simulink model "controller_v10"  (R2020b)
settings: Solver=FixedStepDiscrete  StartTime=0.0  StopTime=inf  RelTol=1e-3
undefined symbols (not defined in the file): ctr, DiscIntNeverNeededParam, flt, IO397, mdl, rbt, rsim, som
libraries: simulink x30, slrealtimeloglib x12, slrealtimeseriallib x5, slrealtimetgmanagement x4, speedgoatlib_fpga_analog_io x4, speedgoatlib_fpga x2, dspfdesign x1, speedgoatlib_fpga_dio x1, slrealtimeutilitieslib x1
(part 2 of 2)

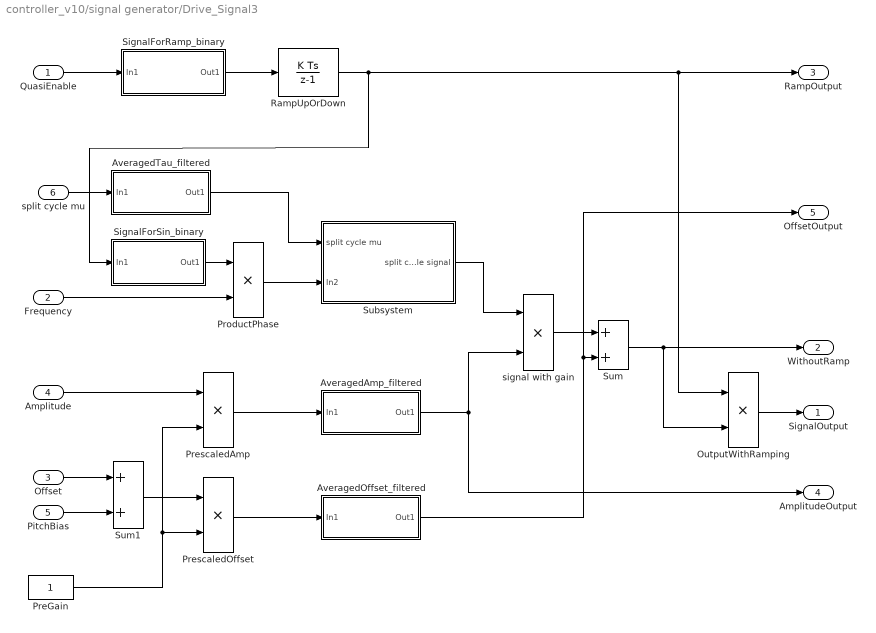
== system controller_v10/signal generator/Drive_Signal3 ==
  QuasiEnable : Inport
  Frequency : Inport  Port=2
  Offset : Inport  Port=3
  Amplitude : Inport  Port=4
  PitchBias : Inport  Port=5
  split cycle mu : Inport  Port=6
  AveragedAmp_filtered : Subsystem
  AveragedOffset_filtered : Subsystem
  AveragedTau_filtered : Subsystem
  OutputWithRamping : Product  RndMeth=Zero
  PreGain : Constant
  PrescaledAmp : Product  RndMeth=Zero
  PrescaledOffset : Product  RndMeth=Zero
  ProductPhase : Product  RndMeth=Zero
  RampUpOrDown : DiscreteIntegrator  gainval=10  SampleTime=-1  LimitOutput=on  UpperSaturationLimit=1  LowerSaturationLimit=0  ICPrevOutput=DiscIntNeverNeededParam  ICPrevScaledInput=DiscIntNeverNeededParam
  SignalForRamp_binary : Subsystem
  SignalForSin_binary : Subsystem
  Subsystem : Subsystem
  Sum : Sum
  Sum1 : Sum
  signal with gain : Product  RndMeth=Zero
  SignalOutput : Outport
  WithoutRamp : Outport  Port=2
  RampOutput : Outport  Port=3
  AmplitudeOutput : Outport  Port=4
  OffsetOutput : Outport  Port=5
  wires:
  PrescaledAmp/1 -> AveragedAmp_filtered/1(In1)
  Sum/1 -> OutputWithRamping/2, WithoutRamp/1
  RampUpOrDown/1 -> RampOutput/1, OutputWithRamping/1, SignalForSin_binary/1(In1)
  QuasiEnable/1 -> SignalForRamp_binary/1(In1)
  SignalForRamp_binary/1(Out1) -> RampUpOrDown/1
  Amplitude/1 -> PrescaledAmp/1
  signal with gain/1 -> Sum/1
  Frequency/1 -> ProductPhase/2
  SignalForSin_binary/1(Out1) -> ProductPhase/1
  ProductPhase/1 -> Subsystem/2(In2)
  AveragedOffset_filtered/1(Out1) -> Sum/2, OffsetOutput/1
  PrescaledOffset/1 -> AveragedOffset_filtered/1(In1)
  PreGain/1 -> PrescaledAmp/2, PrescaledOffset/2
  OutputWithRamping/1 -> SignalOutput/1
  AveragedAmp_filtered/1(Out1) -> signal with gain/2, AmplitudeOutput/1
  Sum1/1 -> PrescaledOffset/1
  Offset/1 -> Sum1/1
  PitchBias/1 -> Sum1/2
  AveragedTau_filtered/1(Out1) -> Subsystem/1(split cycle mu)
  split cycle mu/1 -> AveragedTau_filtered/1(In1)
  Subsystem/1(split cycle signal) -> signal with gain/1

== system controller_v10/signal generator/SignalSaturationLimit ==
  BiasMax : Inport
  SignalRaw : Inport  Port=2
  GainBias : Gain
  MaxOf : MinMax  Function=max  Inputs=2
  MinOf : MinMax  Inputs=2
  ground : Constant
  SignalSatd : Outport
  wires:
  BiasMax/1 -> GainBias/1
  SignalRaw/1 -> MinOf/2
  MinOf/1 -> MaxOf/1
  MaxOf/1 -> SignalSatd/1
  GainBias/1 -> MinOf/1
  ground/1 -> MaxOf/2

== system controller_v10/signal generator/SignalSaturationLimit1 ==
  BiasMax : Inport
  SignalRaw : Inport  Port=2
  GainBias : Gain
  MaxOf : MinMax  Function=max  Inputs=2
  MinOf : MinMax  Inputs=2
  ground : Constant
  SignalSatd : Outport
  wires:
  BiasMax/1 -> GainBias/1
  SignalRaw/1 -> MinOf/2
  MinOf/1 -> MaxOf/1
  MaxOf/1 -> SignalSatd/1
  GainBias/1 -> MinOf/1
  ground/1 -> MaxOf/2

== system controller_v10/signal generator/SignalSaturationLimit2 ==
  BiasMax : Inport
  SignalRaw : Inport  Port=2
  GainBias : Gain
  MaxOf : MinMax  Function=max  Inputs=2
  MinOf : MinMax  Inputs=2
  ground : Constant
  SignalSatd : Outport
  wires:
  BiasMax/1 -> GainBias/1
  SignalRaw/1 -> MinOf/2
  MinOf/1 -> MaxOf/1
  MaxOf/1 -> SignalSatd/1
  GainBias/1 -> MinOf/1
  ground/1 -> MaxOf/2

== system controller_v10/signal generator/SignalSaturationLimit3 ==
  BiasMax : Inport
  SignalRaw : Inport  Port=2
  GainBias : Gain
  MaxOf : MinMax  Function=max  Inputs=2
  MinOf : MinMax  Inputs=2
  ground : Constant
  SignalSatd : Outport
  wires:
  BiasMax/1 -> GainBias/1
  SignalRaw/1 -> MinOf/2
  MinOf/1 -> MaxOf/1
  MaxOf/1 -> SignalSatd/1
  GainBias/1 -> MinOf/1
  ground/1 -> MaxOf/2

== system controller_v10/Adaptive Controller/adaptive system/integrator ==
  note: integrator limit (saturation) needs to be set.
  e : Inport
  torque offset : Inport  Port=2
  thrust_offset : Inport  Port=3
  enable1 : Product  Inputs=**
  initial guess : MATLAB Function  TreatAsAtomicUnit=on
  integrator with sat : DiscreteIntegrator  IntegratorMethod=Integration: Backward Euler  gainval=1  SampleTime=-1  LimitOutput=on  UpperSaturationLimit=ctr.integral.lim.upper  LowerSaturationLimit=ctr.integral.lim.lower  ICPrevOutput=DiscIntNeverNeededParam  ICPrevScaledInput=DiscIntNeverNeededParam
  safety2 : Subsystem
  start ramp : Subsystem
  int_e : Outport
  " torq_off" : Outport  Port=2
  th_off : Outport  Port=3
  wires:
  safety2/1(Out1) -> enable1/2
  enable1/1 -> integrator with sat/1
  start ramp/1(Out1) -> enable1/1
  e/1 -> safety2/1(In1)
  integrator with sat/1 -> initial guess/1(i_e)
  initial guess/1(int_e) -> int_e/1
  initial guess/2(tor_inte) -> " torq_off"/1
  initial guess/3(th_inte) -> th_off/1
  torque offset/1 -> initial guess/2(tor_off)
  thrust_offset/1 -> initial guess/3(th_off)

== system controller_v10/Adaptive Controller/adaptive system/safety1 ==
  In1 : Inport
  Compare To Constant1 : simulink/Logic and Bit Operations/Compare To Constant  relop=<=  const=inf  OutDataTypeStr=uint8
  Switch1 : Switch  Threshold=0.5
  zero1 : Constant  Value=0
  Out1 : Outport
  wires:
  In1/1 -> Switch1/1, Compare To Constant1/1
  Compare To Constant1/1 -> Switch1/2
  zero1/1 -> Switch1/3
  Switch1/1 -> Out1/1

== system controller_v10/Adaptive Controller/adaptive system/safety2 ==
  In1 : Inport
  Compare To Constant1 : simulink/Logic and Bit Operations/Compare To Constant  relop=<=  const=inf  OutDataTypeStr=uint8
  Switch1 : Switch  Threshold=0.5
  zero1 : Constant  Value=0
  Out1 : Outport
  wires:
  In1/1 -> Switch1/1, Compare To Constant1/1
  Compare To Constant1/1 -> Switch1/2
  zero1/1 -> Switch1/3
  Switch1/1 -> Out1/1

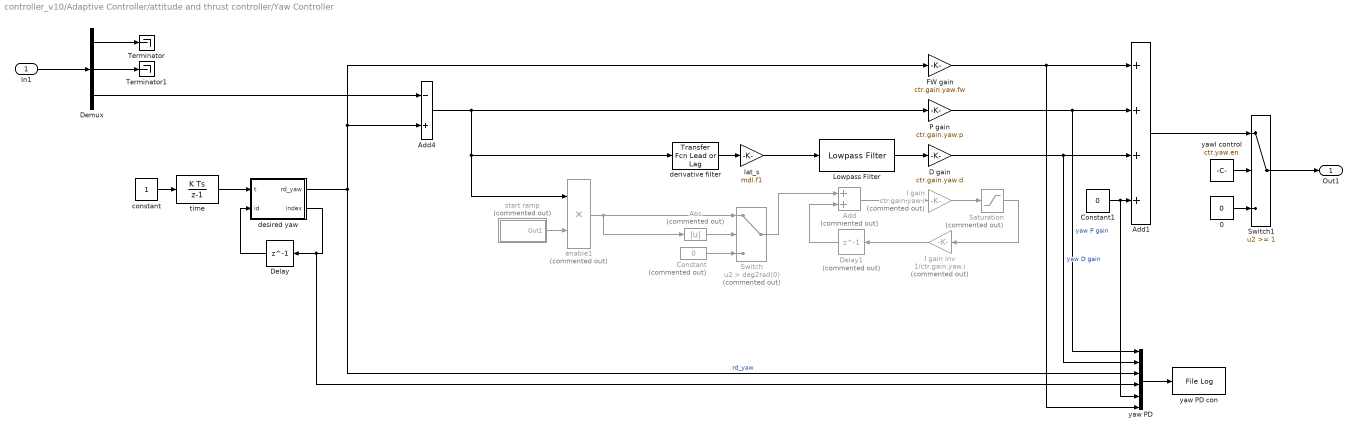
== system controller_v10/Adaptive Controller/attitude and thrust controller/Yaw Controller ==
  In1 : Inport
  0 : Constant  Value=0  SampleTime=-1
  Abs : Abs  Commented=on
  Add : Sum  Commented=on
  Add1 : Sum  Inputs=++++
  Add4 : Sum  Inputs=-+
  Constant : Constant  Commented=on  Value=0
  Constant1 : Constant  Value=0  SampleTime=-1
  D gain : Gain  Gain=ctr.gain.yaw.d
  Delay : Delay  DelayLength=1  InitialCondition=1
  Delay1 : Delay  Commented=on  DelayLength=1
  Demux : Demux  Outputs=3
  FW gain : Gain  Gain=ctr.gain.yaw.fw
  I gain : Gain  Commented=on  Gain=ctr.gain.yaw.i
  I gain inv : Gain  Commented=on  Gain=1/ctr.gain.yaw.i
  Lowpass Filter : dspfdesign/Lowpass Filter  FilterType=FIR  DesignForMinimumOrder=on  FilterOrder=2000  PassbandFrequency=7  StopbandFrequency=90  PassbandRipple=0.5  StopbandAttenuation=75  InheritSampleRate=off  SampleRate=10000  SimulateUsing=Interpreted execution  roundingMode=Floor  coeffsDataTypeStr=fixdt(1,16)
  P gain : Gain  Gain=ctr.gain.yaw.p
  Saturation : Saturate  Commented=on  UpperLimit=ctr.integral.yaw.upper  LowerLimit=ctr.integral.yaw.lower
  Switch : Switch  Commented=on  Criteria=u2 > Threshold  Threshold=deg2rad(0)
  Switch1 : Switch  Threshold=1
  Terminator : Terminator
  Terminator1 : Terminator
  constant : Constant
  derivative filter : simulink/Discrete/Transfer Fcn Lead or Lag  PoleZ=mdl.zf1  ZeroZ=1  ICPrevOutput=0.0  ICPrevInput=0.0  DoSatur=off
      settings: SourceProductBaseCode=SL
  desired yaw : MATLAB Function  TreatAsAtomicUnit=on
  enable1 : Product  Commented=on  Inputs=**
  lat_s : Gain  Gain=mdl.f1
  start ramp : Subsystem  Commented=on
  time : DiscreteIntegrator  gainval=1  SampleTime=-1  UpperSaturationLimit=1  LowerSaturationLimit=0  ICPrevOutput=DiscIntNeverNeededParam  ICPrevScaledInput=DiscIntNeverNeededParam
  yaw PD : Mux  Inputs=6
  yaw PD con : slrealtimeloglib/File Log  decimation=1
      settings: SourceProductBaseCode=XP
  yawl control : Constant  Value=ctr.yaw.en
  Out1 : Outport
  wires:
  Demux/1 -> Terminator/1
  Demux/2 -> Terminator1/1
  Demux/3 -> Add4/1
  0/1 -> Switch1/3
  yawl control/1 -> Switch1/2
  In1/1 -> Demux/1
  Add4/1 -> P gain/1, enable1/1, derivative filter/1
  Switch1/1 -> Out1/1
  derivative filter/1 -> lat_s/1
  Add1/1 -> Switch1/1
  P gain/1 -> yaw PD/1, Add1/2  "yaw P gain"
  D gain/1 -> yaw PD/2, Add1/3  "yaw D gain"
  yaw PD/1 -> yaw PD con/1
  Lowpass Filter/1 -> D gain/1
  lat_s/1 -> Lowpass Filter/1
  constant/1 -> time/1
  time/1 -> desired yaw/1(t)
  desired yaw/1(rd_yaw) -> FW gain/1, Add4/2, yaw PD/3  "rd_yaw"
  desired yaw/2(index) -> yaw PD/4, Delay/1
  Delay/1 -> desired yaw/2(id)
  Saturation/1 -> I gain inv/1
  I gain/1 -> Saturation/1
  enable1/1 -> Switch/1, Abs/1
  Delay1/1 -> Add/2
  Add/1 -> I gain/1
  I gain inv/1 -> Delay1/1
  start ramp/1(Out1) -> enable1/2
  Constant/1 -> Switch/3
  Switch/1 -> Add/1
  Abs/1 -> Switch/2
  FW gain/1 -> yaw PD/6, Add1/1
  Constant1/1 -> yaw PD/5, Add1/4

== system controller_v10/Adaptive Controller/observer/Rotaion ==
  Euler : Inport
  Rotation Matrix : MATLAB Function  TreatAsAtomicUnit=on
  Rotation Matrix1 : MATLAB Function  TreatAsAtomicUnit=on
  filtered derivative : Subsystem
  R : Outport
  Rdot : Outport  Port=2
  Omega : Outport  Port=3
  wires:
  Rotation Matrix/1(R) -> filtered derivative/1(In1), Rotation Matrix1/1(R), R/1
  Euler/1 -> Rotation Matrix/1(euler_angles)
  filtered derivative/1(Out1) -> Rotation Matrix1/2(Rdot), Rdot/1
  Rotation Matrix1/1(w) -> Omega/1

== system controller_v10/Adaptive Controller/observer/lateral observer ==
  XYZ : Inport
  derivative filter : simulink/Discrete/Transfer Fcn Lead or Lag  PoleZ=mdl.zf1  ZeroZ=1  ICPrevOutput=0.0  ICPrevInput=0.0  DoSatur=off
      settings: SourceProductBaseCode=SL
  derivative filter1 : simulink/Discrete/Transfer Fcn Lead or Lag  PoleZ=mdl.zf2  ZeroZ=1  ICPrevOutput=0.0  ICPrevInput=0.0  DoSatur=off
      settings: SourceProductBaseCode=SL
  derivative filter2 : simulink/Discrete/Transfer Fcn Lead or Lag  PoleZ=mdl.zf2  ZeroZ=1  ICPrevOutput=0.0  ICPrevInput=0.0  DoSatur=off
      settings: SourceProductBaseCode=SL
  lat_s : Gain  Gain=mdl.f1
  lat_s2 : Gain  Gain=mdl.f2
  lat_s2_ : Gain  Gain=mdl.f2
  saturation : Subsystem
  r : Outport
  r_dot : Outport  Port=2
  r_dotdot : Outport  Port=3
  wires:
  derivative filter1/1 -> derivative filter2/1
  derivative filter/1 -> lat_s/1
  XYZ/1 -> derivative filter/1, derivative filter1/1, r/1
  derivative filter2/1 -> lat_s2/1
  lat_s/1 -> r_dot/1
  lat_s2/1 -> lat_s2_/1
  lat_s2_/1 -> saturation/1(In1)
  saturation/1(Out1) -> r_dotdot/1

== system controller_v10/Force//Torque to Trajectory Specs/nominal desired voltage/force to voltage (hovering)  ==
  note: apply max voltage limit
  note: known correction from open-loop tests
  force : Inport
  Add : Sum  Inputs=+++
  Constant : Constant  Value=rbt.VM_input1
  Constant1 : Constant  Value=rbt.DV
  Constant2 : Constant  Value=rbt.VM_input2
  MATLAB Function : MATLAB Function  TreatAsAtomicUnit=on
  Product : Product
  Vout : Outport
  wires:
  MATLAB Function/1(Vo) -> Vout/1
  force/1 -> Product/2
  Constant2/1 -> Add/2
  Product/1 -> Add/3
  Add/1 -> MATLAB Function/1(Vi)
  Constant1/1 -> Add/1
  Constant/1 -> Product/1

== system controller_v10/Force//Torque to Trajectory Specs/nominal desired voltage/force to voltage flipping ==
  note: apply max voltage limit
  note: known correction from open-loop tests
  force : Inport
  Add : Sum
  Constant : Constant  Value=rbt.VM2
  Constant1 : Constant  Value=rbt.DV_flip
  MATLAB Function : MATLAB Function  TreatAsAtomicUnit=on
  Product : Product
  Sqrt : Sqrt  SaturateOnIntegerOverflow=on
  Vout : Outport
  wires:
  MATLAB Function/1(Vo) -> Vout/1
  force/1 -> Sqrt/1
  Add/1 -> MATLAB Function/1(Vi)
  Constant1/1 -> Add/1
  Constant/1 -> Product/1
  Product/1 -> Add/2
  Sqrt/1 -> Product/2

== system controller_v10/Measurement manager/safety check system/landing condition ==
  z : Inport
  Add : Sum  Inputs=+--
  SaturatingRamp1 : DiscreteIntegrator  gainval=1  SampleTime=-1  UpperSaturationLimit=1  LowerSaturationLimit=0  ICPrevOutput=DiscIntNeverNeededParam  ICPrevScaledInput=DiscIntNeverNeededParam
  constant : Constant
  constant1 : Constant  Value=2
  constant2 : Constant  Value=mdl.i_delay
  landing_cond : MATLAB Function  TreatAsAtomicUnit=on  SystemSampleTime=mdl.T
  en : Outport
  wires:
  SaturatingRamp1/1 -> Add/1
  constant/1 -> SaturatingRamp1/1
  constant1/1 -> Add/2
  constant2/1 -> Add/3
  Add/1 -> landing_cond/2(time_cond)
  z/1 -> landing_cond/1(alt)
  landing_cond/1(en) -> en/1

== system controller_v10/signal generator/Bias_Signal/AveragedBias ==
  note: To avoid having signal "jump",
      | we want SMOOTH transitions
      | in frequency (i.e., a weighted sum
      | of current freq and freq some delta t ago)
  note: time constant = 0.002sec
  In1 : Inport
  Discrete Transfer Fcn : DiscreteTransferFcn  Numerator=[0.05]  Denominator=[1 -.95]
  Out1 : Outport
  wires:
  In1/1 -> Discrete Transfer Fcn/1
  Discrete Transfer Fcn/1 -> Out1/1

== system controller_v10/signal generator/Bias_Signal/SIgnalForRamp_binary ==
  note: Should output 1 or -1,
      | so signal ramps UP to 1
      | or DOWN to 0.
  In1 : Inport
  Add : Sum  Inputs=+-
  Compare To Zero : simulink/Logic and Bit Operations/Compare To Zero  relop=>  OutDataTypeStr=uint8  ZeroCross=off
  Constant : Constant
  Data Type Conversion : DataTypeConversion  OutDataTypeStr=double
  Gain : Gain  Gain=2
  Out1 : Outport
  wires:
  In1/1 -> Compare To Zero/1
  Compare To Zero/1 -> Data Type Conversion/1
  Gain/1 -> Add/1
  Constant/1 -> Add/2
  Add/1 -> Out1/1
  Data Type Conversion/1 -> Gain/1

== system controller_v10/signal generator/Drive_Signal/AveragedAmp_filtered ==
  note: To avoid having signal "jump",
      | we want SMOOTH transitions
      | in frequency (i.e., a weighted sum
      | of current freq and freq some delta t ago)
  note: time constant 0.002sec
      | for 10kHz samping
  Amplitude : Inport
  Discrete Transfer Fcn : DiscreteTransferFcn  Numerator=[0.05]  Denominator=[1 -.95]
  Out1 : Outport
  wires:
  Amplitude/1 -> Discrete Transfer Fcn/1
  Discrete Transfer Fcn/1 -> Out1/1

== system controller_v10/signal generator/Drive_Signal/SignalForRamp_binary ==
  note: Should output 1 or -1,
      | so signal ramps UP to 1
      | or DOWN to 0.
  In1 : Inport
  Add : Sum  Inputs=+-
  Compare To Zero : simulink/Logic and Bit Operations/Compare To Zero  relop=>  OutDataTypeStr=uint8  ZeroCross=off
  Constant : Constant
  Data Type Conversion : DataTypeConversion  OutDataTypeStr=double
  Gain : Gain  Gain=2
  Out1 : Outport
  wires:
  In1/1 -> Compare To Zero/1
  Compare To Zero/1 -> Data Type Conversion/1
  Gain/1 -> Add/1
  Constant/1 -> Add/2
  Add/1 -> Out1/1
  Data Type Conversion/1 -> Gain/1

== system controller_v10/signal generator/Drive_Signal/SignalForSin_binary ==
  note: We want this to stay "high" for 1
      | second after the actual "enable"
      | is turned off...
  In1 : Inport
  Compare To Zero : simulink/Logic and Bit Operations/Compare To Zero  relop=>  OutDataTypeStr=uint8  ZeroCross=off
  Data Type Conversion : DataTypeConversion  OutDataTypeStr=double
  Out1 : Outport
  wires:
  In1/1 -> Compare To Zero/1
  Compare To Zero/1 -> Data Type Conversion/1
  Data Type Conversion/1 -> Out1/1

== system controller_v10/signal generator/Drive_Signal/Subsystem ==
  note: Amplitude compensation
      | keep the amplitude to be unity
  In2 : Inport
  2pi : Gain  Gain=2*pi
  Add : Sum
  deg to rad : Gain  Gain=pi/180
  first harmonic : Trigonometry  OutputSignalType=real
  omega*t : DiscreteIntegrator  SampleTime=-1  ICPrevOutput=DiscIntNeverNeededParam  ICPrevScaledInput=DiscIntNeverNeededParam
  phase offset : Constant  Value=0
  split cycle signal : Outport
  wires:
  first harmonic/1 -> split cycle signal/1
  In2/1 -> 2pi/1
  2pi/1 -> omega*t/1
  omega*t/1 -> Add/2
  Add/1 -> first harmonic/1
  phase offset/1 -> deg to rad/1
  deg to rad/1 -> Add/1

== system controller_v10/signal generator/Drive_Signal1/AveragedAmp_filtered ==
  note: To avoid having signal "jump",
      | we want SMOOTH transitions
      | in frequency (i.e., a weighted sum
      | of current freq and freq some delta t ago)
  note: time constant 0.002sec
      | for 10kHz samping
  Amplitude : Inport
  Discrete Transfer Fcn : DiscreteTransferFcn  Numerator=[0.05]  Denominator=[1 -.95]
  Out1 : Outport
  wires:
  Amplitude/1 -> Discrete Transfer Fcn/1
  Discrete Transfer Fcn/1 -> Out1/1

== system controller_v10/signal generator/Drive_Signal1/SignalForRamp_binary ==
  note: Should output 1 or -1,
      | so signal ramps UP to 1
      | or DOWN to 0.
  In1 : Inport
  Add : Sum  Inputs=+-
  Compare To Zero : simulink/Logic and Bit Operations/Compare To Zero  relop=>  OutDataTypeStr=uint8  ZeroCross=off
  Constant : Constant
  Data Type Conversion : DataTypeConversion  OutDataTypeStr=double
  Gain : Gain  Gain=2
  Out1 : Outport
  wires:
  In1/1 -> Compare To Zero/1
  Compare To Zero/1 -> Data Type Conversion/1
  Gain/1 -> Add/1
  Constant/1 -> Add/2
  Add/1 -> Out1/1
  Data Type Conversion/1 -> Gain/1

== system controller_v10/signal generator/Drive_Signal1/SignalForSin_binary ==
  note: We want this to stay "high" for 1
      | second after the actual "enable"
      | is turned off...
  In1 : Inport
  Compare To Zero : simulink/Logic and Bit Operations/Compare To Zero  relop=>  OutDataTypeStr=uint8  ZeroCross=off
  Data Type Conversion : DataTypeConversion  OutDataTypeStr=double
  Out1 : Outport
  wires:
  In1/1 -> Compare To Zero/1
  Compare To Zero/1 -> Data Type Conversion/1
  Data Type Conversion/1 -> Out1/1

== system controller_v10/signal generator/Drive_Signal1/Subsystem ==
  In2 : Inport
  2pi : Gain  Gain=2*pi
  Add : Sum
  Constant1 : Constant  Value=0
  SmoothClock : DiscreteIntegrator  SampleTime=-1  ICPrevOutput=DiscIntNeverNeededParam  ICPrevScaledInput=DiscIntNeverNeededParam
  first harmonic : Trigonometry  OutputSignalType=real
  split cycle signal : Outport
  wires:
  SmoothClock/1 -> Add/2
  2pi/1 -> SmoothClock/1
  In2/1 -> 2pi/1
  Add/1 -> first harmonic/1
  Constant1/1 -> Add/1
  first harmonic/1 -> split cycle signal/1

== system controller_v10/signal generator/Drive_Signal2/AveragedAmp_filtered ==
  note: To avoid having signal "jump",
      | we want SMOOTH transitions
      | in frequency (i.e., a weighted sum
      | of current freq and freq some delta t ago)
  note: time constant 0.002sec
      | for 10kHz samping
  In1 : Inport
  Discrete Transfer Fcn : DiscreteTransferFcn  Numerator=[0.05]  Denominator=[1 -.95]
  Out1 : Outport
  wires:
  In1/1 -> Discrete Transfer Fcn/1
  Discrete Transfer Fcn/1 -> Out1/1

== system controller_v10/signal generator/Drive_Signal2/AveragedOffset_filtered ==
  note: To avoid having signal "jump",
      | we want SMOOTH transitions
      | in frequency (i.e., a weighted sum
      | of current freq and freq some delta t ago)
  note: c
  note: time constant 0.02sec
      | for 10kHz samping
  In1 : Inport
  Discrete Transfer Fcn : DiscreteTransferFcn  Numerator=[0.05]  Denominator=[1 -.95]
  Out1 : Outport
  wires:
  In1/1 -> Discrete Transfer Fcn/1
  Discrete Transfer Fcn/1 -> Out1/1

== system controller_v10/signal generator/Drive_Signal2/AveragedTau_filtered ==
  note: To avoid having signal "jump",
      | we want SMOOTH transitions
      | in frequency (i.e., a weighted sum
      | of current freq and freq some delta t ago)
  note: time constant 0.002sec
      | for 10kHz samping
  In1 : Inport
  Discrete Transfer Fcn : DiscreteTransferFcn  Numerator=[0.05]  Denominator=[1, -0.95]
  Out1 : Outport
  wires:
  In1/1 -> Discrete Transfer Fcn/1
  Discrete Transfer Fcn/1 -> Out1/1

== system controller_v10/signal generator/Drive_Signal2/SignalForRamp_binary ==
  note: Should output 1 or -1,
      | so signal ramps UP to 1
      | or DOWN to 0.
  In1 : Inport
  Add : Sum  Inputs=+-
  Compare To Zero : simulink/Logic and Bit Operations/Compare To Zero  relop=>  OutDataTypeStr=uint8  ZeroCross=off
  Constant : Constant
  Data Type Conversion : DataTypeConversion  OutDataTypeStr=double
  Gain : Gain  Gain=2
  Out1 : Outport
  wires:
  In1/1 -> Compare To Zero/1
  Compare To Zero/1 -> Data Type Conversion/1
  Gain/1 -> Add/1
  Constant/1 -> Add/2
  Add/1 -> Out1/1
  Data Type Conversion/1 -> Gain/1

== system controller_v10/signal generator/Drive_Signal2/SignalForSin_binary ==
  note: We want this to stay "high" for 1
      | second after the actual "enable"
      | is turned off...
  In1 : Inport
  Compare To Zero : simulink/Logic and Bit Operations/Compare To Zero  relop=>  OutDataTypeStr=uint8  ZeroCross=off
  Data Type Conversion : DataTypeConversion  OutDataTypeStr=double
  Out1 : Outport
  wires:
  In1/1 -> Compare To Zero/1
  Compare To Zero/1 -> Data Type Conversion/1
  Data Type Conversion/1 -> Out1/1

== system controller_v10/signal generator/Drive_Signal2/Subsystem ==
  note: positive value pushes the left wing forward
  split cycle mu : Inport
  In2 : Inport  Port=2
  1-mu : Sum  Inputs=+-
  2f : Gain  Gain=2
  2nd harmonic : Trigonometry  OutputSignalType=real
  2pi : Gain  Gain=2*pi
  Abs1 : Abs
  Add : Sum
  Constant : Constant
  combined sines : Sum
  deg to rad : Gain  Gain=pi/180
  f : Gain  Gain=-1
  first harmonic : Trigonometry  OutputSignalType=real
  omega*t : DiscreteIntegrator  SampleTime=-1  ICPrevOutput=DiscIntNeverNeededParam  ICPrevScaledInput=DiscIntNeverNeededParam
  phase offset : Constant  Value=180
  signal with gain1 : Product  RndMeth=Zero
  signal with gain2 : Product  RndMeth=Zero
  split cycle signal : Outport
  wires:
  2f/1 -> 2nd harmonic/1
  first harmonic/1 -> signal with gain1/2
  Constant/1 -> 1-mu/1
  split cycle mu/1 -> f/1, Abs1/1
  1-mu/1 -> signal with gain1/1
  2nd harmonic/1 -> signal with gain2/2
  signal with gain1/1 -> combined sines/1
  signal with gain2/1 -> combined sines/2
  combined sines/1 -> split cycle signal/1
  f/1 -> signal with gain2/1
  Abs1/1 -> 1-mu/2
  In2/1 -> 2pi/1
  2pi/1 -> omega*t/1
  omega*t/1 -> Add/2
  Add/1 -> first harmonic/1, 2f/1
  phase offset/1 -> deg to rad/1
  deg to rad/1 -> Add/1

== system controller_v10/signal generator/Drive_Signal3/AveragedAmp_filtered ==
  note: To avoid having signal "jump",
      | we want SMOOTH transitions
      | in frequency (i.e., a weighted sum
      | of current freq and freq some delta t ago)
  note: time constant 0.002sec
      | for 10kHz samping
  In1 : Inport
  Discrete Transfer Fcn : DiscreteTransferFcn  Numerator=[0.05]  Denominator=[1 -.95]
  Out1 : Outport
  wires:
  In1/1 -> Discrete Transfer Fcn/1
  Discrete Transfer Fcn/1 -> Out1/1

== system controller_v10/signal generator/Drive_Signal3/AveragedOffset_filtered ==
  note: To avoid having signal "jump",
      | we want SMOOTH transitions
      | in frequency (i.e., a weighted sum
      | of current freq and freq some delta t ago)
  note: c
  note: time constant 0.02sec
      | for 10kHz samping
  In1 : Inport
  Discrete Transfer Fcn : DiscreteTransferFcn  Numerator=[0.05]  Denominator=[1 -.95]
  Out1 : Outport
  wires:
  In1/1 -> Discrete Transfer Fcn/1
  Discrete Transfer Fcn/1 -> Out1/1

== system controller_v10/signal generator/Drive_Signal3/AveragedTau_filtered ==
  note: To avoid having signal "jump",
      | we want SMOOTH transitions
      | in frequency (i.e., a weighted sum
      | of current freq and freq some delta t ago)
  note: time constant 0.002sec
      | for 10kHz samping
  In1 : Inport
  Discrete Transfer Fcn : DiscreteTransferFcn  Numerator=[0.05]  Denominator=[1 -.95]
  Out1 : Outport
  wires:
  In1/1 -> Discrete Transfer Fcn/1
  Discrete Transfer Fcn/1 -> Out1/1

== system controller_v10/signal generator/Drive_Signal3/SignalForRamp_binary ==
  note: Should output 1 or -1,
      | so signal ramps UP to 1
      | or DOWN to 0.
  In1 : Inport
  Add : Sum  Inputs=+-
  Compare To Zero : simulink/Logic and Bit Operations/Compare To Zero  relop=>  OutDataTypeStr=uint8  ZeroCross=off
  Constant : Constant
  Data Type Conversion : DataTypeConversion  OutDataTypeStr=double
  Gain : Gain  Gain=2
  Out1 : Outport
  wires:
  In1/1 -> Compare To Zero/1
  Compare To Zero/1 -> Data Type Conversion/1
  Gain/1 -> Add/1
  Constant/1 -> Add/2
  Add/1 -> Out1/1
  Data Type Conversion/1 -> Gain/1

== system controller_v10/signal generator/Drive_Signal3/SignalForSin_binary ==
  note: We want this to stay "high" for 1
      | second after the actual "enable"
      | is turned off...
  In1 : Inport
  Compare To Zero : simulink/Logic and Bit Operations/Compare To Zero  relop=>  OutDataTypeStr=uint8  ZeroCross=off
  Data Type Conversion : DataTypeConversion  OutDataTypeStr=double
  Out1 : Outport
  wires:
  In1/1 -> Compare To Zero/1
  Compare To Zero/1 -> Data Type Conversion/1
  Data Type Conversion/1 -> Out1/1

== system controller_v10/signal generator/Drive_Signal3/Subsystem ==
  split cycle mu : Inport
  In2 : Inport  Port=2
  1-mu : Sum  Inputs=+-
  2f : Gain  Gain=2
  2nd harmonic : Trigonometry  OutputSignalType=real
  2pi : Gain  Gain=2*pi
  Abs1 : Abs
  Constant : Constant
  SmoothClock : DiscreteIntegrator  SampleTime=-1  ICPrevOutput=DiscIntNeverNeededParam  ICPrevScaledInput=DiscIntNeverNeededParam
  combined sines : Sum
  f : Gain
  first harmonic : Trigonometry  OutputSignalType=real
  signal with gain1 : Product  RndMeth=Zero
  signal with gain2 : Product  RndMeth=Zero
  split cycle signal : Outport
  wires:
  SmoothClock/1 -> first harmonic/1, 2f/1
  2f/1 -> 2nd harmonic/1
  2pi/1 -> SmoothClock/1
  first harmonic/1 -> signal with gain1/2
  Constant/1 -> 1-mu/1
  split cycle mu/1 -> f/1, Abs1/1
  1-mu/1 -> signal with gain1/1
  2nd harmonic/1 -> signal with gain2/2
  signal with gain1/1 -> combined sines/1
  signal with gain2/1 -> combined sines/2
  combined sines/1 -> split cycle signal/1
  In2/1 -> 2pi/1
  f/1 -> signal with gain2/1
  Abs1/1 -> 1-mu/2

== system controller_v10/Adaptive Controller/adaptive system/integrator/safety2 ==
  In1 : Inport
  Compare To Constant1 : simulink/Logic and Bit Operations/Compare To Constant  relop=<=  const=inf  OutDataTypeStr=uint8
  Switch1 : Switch  Threshold=0.5
  zero1 : Constant  Value=0
  Out1 : Outport
  wires:
  In1/1 -> Switch1/1, Compare To Constant1/1
  Compare To Constant1/1 -> Switch1/2
  zero1/1 -> Switch1/3
  Switch1/1 -> Out1/1

== system controller_v10/Adaptive Controller/adaptive system/integrator/start ramp ==
  0.8 : Constant  Value=mdl.s_delay
  2 : Constant  Value=mdl.i_delay
  Add1 : Sum
  Add2 : Sum  Inputs=+-
  Compare To Zero : simulink/Logic and Bit Operations/Compare To Zero  relop=>  OutDataTypeStr=uint8  ZeroCross=off
  Data Type Conversion : DataTypeConversion
  constant : Constant
  counter : DiscreteIntegrator  gainval=1  SampleTime=-1  UpperSaturationLimit=1  LowerSaturationLimit=0  ICPrevOutput=DiscIntNeverNeededParam  ICPrevScaledInput=DiscIntNeverNeededParam
  saturation ramp : DiscreteIntegrator  gainval=5  SampleTime=-1  LimitOutput=on  UpperSaturationLimit=1  LowerSaturationLimit=-1  ICPrevOutput=DiscIntNeverNeededParam  ICPrevScaledInput=DiscIntNeverNeededParam
  Out1 : Outport
  wires:
  constant/1 -> counter/1
  2/1 -> Add1/1
  0.8/1 -> Add1/2
  counter/1 -> Add2/1
  Add1/1 -> Add2/2
  Add2/1 -> Compare To Zero/1
  Compare To Zero/1 -> Data Type Conversion/1
  saturation ramp/1 -> Out1/1
  Data Type Conversion/1 -> saturation ramp/1

== system controller_v10/Adaptive Controller/attitude and thrust controller/Yaw Controller/start ramp ==
  0.8 : Constant  Value=0.01
  2 : Constant  Value=mdl.i_delay
  Add1 : Sum
  Add2 : Sum  Inputs=+-
  Compare To Zero : simulink/Logic and Bit Operations/Compare To Zero  relop=>  OutDataTypeStr=uint8  ZeroCross=off
  Data Type Conversion : DataTypeConversion
  constant : Constant
  counter : DiscreteIntegrator  gainval=1  SampleTime=-1  UpperSaturationLimit=1  LowerSaturationLimit=0  ICPrevOutput=DiscIntNeverNeededParam  ICPrevScaledInput=DiscIntNeverNeededParam
  saturation ramp : DiscreteIntegrator  gainval=5  SampleTime=-1  LimitOutput=on  UpperSaturationLimit=1  LowerSaturationLimit=-1  ICPrevOutput=DiscIntNeverNeededParam  ICPrevScaledInput=DiscIntNeverNeededParam
  Out1 : Outport
  wires:
  constant/1 -> counter/1
  2/1 -> Add1/1
  0.8/1 -> Add1/2
  counter/1 -> Add2/1
  Add1/1 -> Add2/2
  Add2/1 -> Compare To Zero/1
  Compare To Zero/1 -> Data Type Conversion/1
  saturation ramp/1 -> Out1/1
  Data Type Conversion/1 -> saturation ramp/1

== system controller_v10/Adaptive Controller/observer/Rotaion/filtered derivative ==
  In1 : Inport
  att_s : Gain  Gain=mdl.f1
  filtered derivative : simulink/Discrete/Transfer Fcn Lead or Lag  PoleZ=mdl.zf1  ZeroZ=1  ICPrevOutput=0.0  ICPrevInput=0.0  DoSatur=off
      settings: SourceProductBaseCode=SL
  low pass3 : DiscreteTransferFcn  Numerator=mdl.vlp.n  Denominator=mdl.vlp.d
  Out1 : Outport
  wires:
  filtered derivative/1 -> low pass3/1
  att_s/1 -> filtered derivative/1
  In1/1 -> att_s/1
  low pass3/1 -> Out1/1

== system controller_v10/Adaptive Controller/observer/lateral observer/saturation ==
  In1 : Inport
  MinMax2 : MinMax  Inputs=2
  MinMax3 : MinMax  Function=max  Inputs=2
  lw1 : Constant  Value=-mdl.fd_lim
  up1 : Constant  Value=mdl.fd_lim
  Out1 : Outport
  wires:
  In1/1 -> MinMax2/2
  up1/1 -> MinMax2/1
  lw1/1 -> MinMax3/1
  MinMax2/1 -> MinMax3/2
  MinMax3/1 -> Out1/1

== matlab function controller_v10/Adaptive Controller/adaptive setpoint rd ==
  data: rd output; rd_d output; rd_dd output; rd_ddd output; rd_dddd output; time input; r input; r_d input; landing input; som_ph input; ctr parameter; som parameter; mdl parameter
function [rd,rd_d,rd_dd,rd_ddd,rd_dddd] = fcn(time, r, r_d, landing,som_ph, ctr, som, mdl)
%#codegen

rd = [ctr.setpoint.x; ctr.setpoint.y; ctr.setpoint.z];
rd_d = zeros(3,1);
rd_dd = zeros(3,1);
rd_ddd = zeros(3,1);
rd_dddd = zeros(3,1);

if time <= mdl.i_delay
    rd_z = 0;
    rd   = [ctr.setpoint.x; ctr.setpoint.y; rd_z];
end

% takeoff
if ctr.takeoff.en
    if time > mdl.i_delay && time < (mdl.i_delay+ctr.takeoff.time)
        rd_z = ctr.takeoff.height + (((ctr.setpoint.z-ctr.takeoff.height)/ctr.takeoff.time)*(time-mdl.i_delay));
        if rd_z > ctr.setpoint.z
            rd_z = ctr.setpoint.z;
        end
        rd   = [ctr.setpoint.x; ctr.setpoint.y; rd_z];
    end
end

% planned landing 
if ctr.landing.en
    if time > (mdl.rt-ctr.landing.time)
        rd_z = ctr.setpoint.z-(((ctr.setpoint.z-ctr.landing.height)/ctr.landing.time)*(time-mdl.rt+ctr.landing.time));
        if rd_z < ctr.landing.height
            rd_z = ctr.landing.height;
        end
        rd   = [ctr.setpoint.x; ctr.setpoint.y; rd_z];
    end
end

% forced landing
if landing
    rd_z = 0.02;
    rd   = [ctr.setpoint.x; ctr.setpoint.y; rd_z];
end


% somersault
if som.en
    if time > som.t_start + som.t_rise + som.t_acc + som.t_dcc + som.t_rec
        % % afterwards 
        %dt = som.t_start + som.t_rise + som.t_acc + som.t_dcc + som.t_rec - time;
        %rd = rd + dt*(r-rd);
    elseif time > som.t_start + som.t_rise + som.t_acc + som.t_dcc
        % recovery
        dt = som.t_start + som.t_rise + som.t_acc + som.t_dcc + som.t_rec - time;
        rd = rd + (dt/som.t_rec)*(r-rd);
        rd_d = rd_d + 0.5*(dt/som.t_rec)*(r_d-rd_d);
        rd(1) = min(max(rd(1),-0.25),0.25); % 25 cm envelope
        rd(2) = min(max(rd(2),-0.25),0.25); % 25 cm envelope
        rd(3) = max(rd(3),0.02); % min altitude setpoint.
    end
end


end

== matlab function controller_v10/Force//Torque to Trajectory Specs/nominal desired voltage/force to voltage (hovering) /MATLAB Function ==
  data: Vi input; Vo output; mdl parameter
function Vo = fcn(Vi,mdl)
%old script
% if max(Vi)>mdl.max_v
%     Vo = Vi * mdl.max_v/max(Vi);
%     % scale down all votages if one exceeds the max limit.
% else
%     Vo = Vi;
% end

%new change (modify max_v to a vector so each DEA has its own max)
% scale_down_ratio_vec = Vi ./ mdl.max_v_vec;
% scale_down_ratio = max(scale_down_ratio_vec);
% bool_scale_down = scale_down_ratio>1;
% 
% if bool_scale_down
%    Vo = Vi/scale_down_ratio;
% else
%    Vo = Vi; 
% end

min_v_vec = mdl.hovering_vec -150;
scale_down_ratio_vec = (Vi-min_v_vec)./(mdl.max_v_vec-min_v_vec);

scale_down_ratio = max(scale_down_ratio_vec);
bool_scale_down = scale_down_ratio>1;

if bool_scale_down
    Vo = min_v_vec + (Vi - min_v_vec)./scale_down_ratio;	
else
	  Vo = Vi; 
end


%extra layer of safety
for i=1:length(Vo)
	Vo(i) = min(Vo(i),mdl.max_v_vec(i));
end

== matlab function controller_v10/Adaptive Controller/somersault_phase ==
  data: som_phase output; time input; mdl parameter; som parameter
function som_phase  = fcn(time, mdl, som)
%#codegen

som_phase = 0;  % during a normal flight
if som.en
    if time > som.t_start + som.t_rise + som.t_acc + som.t_dcc + som.t_rec
        som_phase = 0;  % afterwards
    elseif time > som.t_start + som.t_rise + som.t_acc + som.t_dcc
        som_phase = 4;  % recovery
    elseif time > som.t_start + som.t_rise + som.t_acc
        som_phase = 3;  % rolling, second half.
    elseif time > som.t_start + som.t_rise
        som_phase = 2;  % rolling, first half.
    elseif time > som.t_start
        som_phase = 1;  % gaining altitude
    end
end

== matlab function controller_v10/Force//Torque to Trajectory Specs/nominal desired voltage/force to voltage flipping/MATLAB Function ==
  data: Vi input; Vo output; mdl parameter
function Vo = fcn(Vi,mdl)
%old script
% if max(Vi)>mdl.max_v
%     Vo = Vi * mdl.max_v/max(Vi);
%     % scale down all votages if one exceeds the max limit.
% else
%     Vo = Vi;
% end

%new change (modify max_v to a vector so each DEA has its own max)
scale_down_ratio_vec = Vi ./ mdl.max_v_vec;
scale_down_ratio = max(scale_down_ratio_vec);
bool_scale_down = scale_down_ratio>1;

if bool_scale_down
   Vo = Vi/scale_down_ratio;
else
   Vo = Vi; 
end

== matlab function controller_v10/smothing/smoothing ==
  data: time input; out_amp output; amp input; amp2 input; som parameter
function out_amp  = fcn(time,amp,amp2,som)
%#codegen

alp = 1;
if time > som.t_start + som.t_rise + som.t_acc + som.t_dcc + som.t_rec
    alp = 1;  % afterwards
elseif time > som.t_start
    alp = som.filter.alp;
end
% set en = 0 if the robot goes out of the safe envelope.
out_amp = som.filter.alp*amp + (1-som.filter.alp)*amp2;

== matlab function controller_v10/Adaptive Controller/saturation ==
  data: x_roll input; X_roll output size=1; y_pitch input; z_yaw input; Y_pitch output size=1; Z_yaw output size=1; Th input; Force output size=1; rbt parameter; ctr parameter; som_phase input; som parameter
function [X_roll, Y_pitch, Z_yaw, Force] = fcn(x_roll, y_pitch, z_yaw, Th, rbt, ctr, som_phase, som)
%#codegen

X_roll = max(min(x_roll, ctr.lim.taux), -ctr.lim.taux);
%X_roll = x_roll;
Y_pitch = max(min(y_pitch, ctr.lim.tauy), -ctr.lim.tauy);
%Y_pitch = y_pitch;
Z_yaw = max(min(z_yaw, ctr.lim.tauz), -ctr.lim.tauz);

Force = Th*rbt.m;

% F is already checked for saturation, but still needs to be converted into
% Newton

%% Roll torque management (somersault)
if som_phase == 2
    X_roll = som.roll_mag; % torque in SI
    Y_pitch = 0;  % to turn of the pitch control
elseif som_phase == 3
    X_roll = -som.roll_mag; % torque in SI
    Y_pitch = 0;  % to turn of the pitch control
end
    
%% Thrust management
% thrust is not controlled during the flipping maneuver (the output here will be overridden in the mapping).

== matlab function controller_v10/Force//Torque to Trajectory Specs/force//torque to module thrust/mapping scheme (flipping compataible) ==
  data: time input; module_f output; inputs input; rbt parameter; som parameter; mdl parameter
function module_f  = fcn(time, inputs, rbt, som, mdl)

% somersault
if som.en
    if time > som.t_start + som.t_rise + som.t_acc + som.t_dcc+som.t_rec % after recovery
        %
    elseif time > som.t_start + som.t_rise + som.t_acc + som.t_dcc % recovery
        %inputs(1) = rbt.m*(mdl.g*(som.thrust_f+0.2));
    elseif time > som.t_start + som.t_rise % rolling, first half+second half.
        % priortize the roll torque and ensure non-negative forces.
        inputs(1) = 0;
    elseif time > som.t_start
        inputs(1) = rbt.m*(mdl.g*som.thrust_f); % during the t rise.                
    end
end

% torque/thrust to unit force mapping
if rbt.til == 0
    module_f = rbt.Apinv * inputs(1:3); % original mapping
elseif rbt.til > 0
    module_f = rbt.A2inv * inputs;
else
    module_f = [0 0 0 0]';
end

% safety
if min(module_f) < 0
    module_f = module_f - min(module_f); % this ensure positive module forces
end

end

== matlab function controller_v10/Adaptive Controller/adaptive system/integrator/initial guess ==
  data: i_e input; int_e output; tor_off input; th_off input; tor_inte output; th_inte output; ctr parameter; rbt parameter; mdl parameter
function [int_e, tor_inte, th_inte] = fcn(i_e, tor_off, th_off, ctr, rbt, mdl)
%#codegen

tor_inte = zeros(3,1);
int_e    = zeros(4,1);

int_e(1) = i_e(1)+tor_off(1);
int_e(2) = i_e(2)+tor_off(2);
int_e(3) = i_e(3)+tor_off(3);
int_e(4) = i_e(4)+th_off;

tor_inte(1) = int_e(1)*ctr.gain.ati*rbt.ixx/mdl.g;
tor_inte(2) = int_e(2)*ctr.gain.ati*rbt.iyy/mdl.g;
tor_inte(3) = 0;

th_inte     = int_e(4)*ctr.gain.ali;

== matlab function controller_v10/Phantom trigger/start at one ==
  data: time input; trigger output
function trigger = fcn(time)
%#codegen
trigger = 0;
if time > 1
   trigger = 1; 
end
if time > 2
   trigger = 0; 
end

== matlab function controller_v10/Measurement manager/safety check system/envelope check ==
  data: x input; en output; y input; z input; ctr parameter
function en  = fcn(x,y,z, ctr)

if abs(x)>ctr.safety.enableZone.xmax || abs(y)>ctr.safety.enableZone.ymax || abs(z)>ctr.safety.enableZone.zmax
    en = 0;
else
    en = 1;
end

end

== matlab function controller_v10/Dynamic Sim/conditioning ==
  data: Rout output; Rin input; eu output
function [Rout, eu]  = fcn(Rin)
%#codegen
Rm = [Rin(1:3)./norm(Rin(1:3)),Rin(4:6)./norm(Rin(4:6)),Rin(7:9)./norm(Rin(7:9))];
% conditioning on orthogonality.
Rout = [Rm(:,1);Rm(:,2);Rm(:,3)];

% euler angles
euy = asin(min(max(Rm(1,3),-1),1));
eux = atan2(-Rm(2,3),Rm(3,3));
euz = atan2(-Rm(1,2),Rm(1,1));
%euz=acos(min(max(Rm(1,1)/cos(euy),-1),1));
%eux=acos(min(max(Rm(3,3)/cos(euy),-1),1));
eu = [eux;euy;euz];
% not being very careful with singularities.

== matlab function controller_v10/Force//Torque to Trajectory Specs/nominal desired voltage/map_selection ==
  data: hover_map output; time input; mdl parameter; som parameter
function hover_map  = fcn(time, mdl, som)
%#codegen

hover_map = 1;  % during a normal flight
if som.en
    if time > som.t_start + som.t_rise + som.t_acc + som.t_dcc
        hover_map = 1;  % afterwards
    elseif time > som.t_start + som.t_rise
    %elseif time > som.t_start + som.t_rise 
        hover_map = 0;  % 
    end
end

== matlab function controller_v10/Dynamic Sim/rigid body dynamics sim ==
  data: dv output double size=3; mforces input double; dR output double size=9; dw output double size=3; v input; R input; w input; rbt parameter; mdl parameter; disturbance input; rsim parameter
function [dv, dR, dw]  = fcn(mforces,v,R,w,rbt,mdl,disturbance, rsim)
%#codegen

% noiseless
% no damping
% rbt_A_temp = [rbt.A; 0.015 -0.015 0.015 -0.015];
rbt_A_temp = rbt.A2;
% inputs = rbt.A * mforces(:);
inputs = rbt_A_temp * mforces(:);
thrust = inputs(1);
% torque = [inputs(2);inputs(3);0];
torque = [inputs(2);inputs(3);inputs(4)];
%R = R(:);
%w = w(:);
dv = R(7:9)*thrust/rbt.m - [0;0;mdl.g] + disturbance(1:3);

dw = diag([rsim.rbt.ixx, rsim.rbt.iyy, rsim.rbt.izz]) \ ( (torque) - cross(w,diag([rsim.rbt.ixx, rsim.rbt.iyy, rsim.rbt.izz])*w)+ disturbance(4:6) ) ;
dR1 = R(4:6)*w(3)-R(7:9)*w(2);
dR2 = R(7:9)*w(1)-R(1:3)*w(3);
dR3 = R(1:3)*w(2)-R(4:6)*w(1);
dR = [dR1;dR2;dR3];
%dv = zeros(3,1);
%dw = zeros(3,1);
%dR = zeros(9,1);

== matlab function controller_v10/Adaptive Controller/attitude and thrust controller/Yaw Controller/desired yaw ==
  data: t input; id input; rd_yaw output; ctr parameter; index output; mdl parameter
function [rd_yaw, index] = fcn(t,id,ctr,mdl)

if ctr.yaw.dy.en
    
    if id > 1
        t_cum = sum(ctr.yaw.dy.duration(1:id-1))+sum(ctr.yaw.dy.trans(1:id-1));
    else
        t_cum = 0;
    end

    if t > mdl.i_delay + t_cum && t <= mdl.i_delay + t_cum + ctr.yaw.dy.duration(id)
        rd_yaw = ctr.yaw.dy.angle(id);
    elseif t > mdl.i_delay + t_cum + ctr.yaw.dy.duration(id) && t < mdl.i_delay + t_cum + ctr.yaw.dy.duration(id) + ctr.yaw.dy.trans(id)
        rd_yaw = ctr.yaw.dy.angle(id) + (ctr.yaw.dy.angle(id+1)-ctr.yaw.dy.angle(id))/ctr.yaw.dy.trans(id)*(t-mdl.i_delay-t_cum-ctr.yaw.dy.duration(id));
    elseif t >= mdl.i_delay + t_cum + ctr.yaw.dy.duration(id) + ctr.yaw.dy.trans(id)
        rd_yaw = ctr.yaw.dy.angle(id+1);
        id = id + 1;
    else
        rd_yaw = 0;
    end

else
    
    rd_yaw = ctr.setpoint.yaw;
    
end

index = id;
    
end

== matlab function controller_v10/Measurement manager/safety check system/voltage check ==
  data: voltage input; en output; ctr parameter
function en  = fcn(voltage, ctr)

if sum(voltage>ctr.safety.volt) > 0
    en = 0;
else
    en = 1;
end

end

== matlab function controller_v10/Measurement manager/envelope//voltage check ==
  data: x input; keep_flying output size=1; y input; z input; ctr parameter
function keep_flying  = fcn(x,y,z,ctr)

if abs(x)>ctr.safety.land.xmax || abs(y)>ctr.safety.land.ymax || abs(z)>ctr.safety.land.zmax
    keep_flying = 0;
% elseif voltage(1) > ctr.safety.land.volt
%     keep_flying = 0;    
else
    keep_flying = 1;
end

end

== matlab function controller_v10/Measurement manager/MATLAB Function ==
  data: keep_flying input; landing_in input; landing_out output size=1; cum_in input; cum_out output size=1; ctr parameter; mdl parameter
function [landing_out, cum_out] = fcn(keep_flying, landing_in, cum_in, ctr, mdl)

if keep_flying == 0
    cum_out = cum_in + mdl.T;
else
    cum_out = 0;
end

if cum_out > ctr.safety.land.T || landing_in == 1
    landing_out = 1;
else 
    landing_out = 0;
end

end

== matlab function controller_v10/Measurement manager/voltage check ==
  data: voltage input; keep_flying output size=1; ctr parameter
function keep_flying  = fcn(voltage, ctr)

% if voltage(1)>ctr.safety.land.volt || voltage(2)>ctr.safety.land.volt || voltage(3)>ctr.safety.land.volt || voltage(4)>ctr.safety.land.volt

if sum(voltage>ctr.safety.land.volt)>0
    keep_flying = 0;
else
    keep_flying = 1;
end

end

== matlab function controller_v10/Measurement manager/safety check system/MATLAB Function ==
  data: keep_flying input; en_in input; en_out output size=1; cum_in input; cum_out output size=1; ctr parameter; mdl parameter
function [en_out, cum_out] = fcn(keep_flying, en_in, cum_in, ctr, mdl)

if keep_flying == 0
    cum_out = cum_in + mdl.T;
else
    cum_out = 0;
end

if cum_out > ctr.safety.T || en_in == 0
    en_out = 0;
else 
    en_out = 1;
end

end

== matlab function controller_v10/Adaptive Controller/observer/Rotaion/Rotation Matrix1 ==
  data: R input; Rdot input; w output
function w  = fcn(R,Rdot)
%#codegen
w = zeros(3,1);
w(1) = R(3)*Rdot(2) + R(6)*Rdot(5) + R(9)*Rdot(8);
w(2) = R(1)*Rdot(3) + R(4)*Rdot(6) + R(7)*Rdot(9);
w(3) = R(2)*Rdot(1) + R(5)*Rdot(4) + R(8)*Rdot(7);

== matlab function controller_v10/Adaptive Controller/attitude and thrust controller/Attitude Controleller ==
  data: r input; torque_x output size=1; r_dot input; r_dotdot input; R input; Omega input; rd input; rd_d input; rd_dd input; rd_ddd input; rd_dddd input; int_e input; ctr parameter; rbt parameter; torque_y output size=1; torque_z output size=1; att_e output size=3; mdl parameter
 function [torque_x, torque_y, torque_z, att_e] = fcn(r, r_dot, r_dotdot, R, Omega, rd,rd_d,rd_dd,rd_ddd,rd_dddd, int_e, ctr, rbt, mdl)
%#codegen

%% init
R11 = R(1);
R12 = R(2);
R13 = R(3);
R21 = R(4);
R22 = R(5);
R23 = R(6);
R31 = R(7);
R32 = R(8);
R33 = R(9);
R1 = [R11; R21; R31];     % unit (column) vector
R2 = [R12; R22; R32];
R3 = [R13; R23; R33];
wx = Omega(1);
wy = Omega(2);
wz = Omega(3);

Dr = r-rd;
Dr_dot = r_dot-rd_d;

torque_x = -dot(R2,rd_dddd) - ...
    ctr.gain.at3*( mdl.g*wx+dot(R2,rd_ddd) ) - ...
    ctr.gain.at2*( dot(R2,mdl.g*[0;0;1]+rd_dd) ) + ...
    ctr.gain.at1*( dot(R2,Dr_dot) ) + ...
    ctr.gain.at0*( dot(R2,Dr) ) + ...
    ctr.gain.ati*( int_e(1) );
torque_x = torque_x*rbt.ixx/mdl.g;

torque_y = dot(R1,rd_dddd) - ...
    ctr.gain.at3*( mdl.g*wy-dot(R1,rd_ddd) ) - ...
    ctr.gain.at2*( dot(R1,-mdl.g*[0;0;1]-rd_dd) ) - ...
    ctr.gain.at1*( dot(R1,Dr_dot) ) - ...
    ctr.gain.at0*( dot(R1,Dr) ) + ...
    ctr.gain.ati*( int_e(2) );

torque_y = torque_y*rbt.iyy/mdl.g;

torque_z = 0;           % no yaw control

att_e = -[-dot(R2,Dr);dot(R1,Dr);0];

== matlab function controller_v10/Measurement manager/safety check system/landing condition/landing_cond ==
  data: alt input; en output; time_cond input; ctr parameter
function en = fcn(alt,time_cond,ctr)
%#codegen
if ( (time_cond<0) | (alt>ctr.landing.height) )
    en = 1;
else
    en = 0;
end
en=1;
end
% this lands the robot if the flight time is more than mdl.i_delay+2 and
% the robot is still on the ground.

== matlab function controller_v10/Adaptive Controller/observer/Rotaion/Rotation Matrix ==
  data: euler_angles input; R output
function R = fcn(euler_angles)
%#codegen

eu_x = euler_angles(1);
eu_y = euler_angles(2);
eu_z = euler_angles(3);

R = [cos(eu_y)*cos(eu_z); -cos(eu_y)*sin(eu_z); sin(eu_y); ...
    cos(eu_x)*sin(eu_z)+sin(eu_x)*sin(eu_y)*cos(eu_z); cos(eu_x)*cos(eu_z)-sin(eu_x)*sin(eu_y)*sin(eu_z); -sin(eu_x)*cos(eu_y); ...
    sin(eu_x)*sin(eu_z)-cos(eu_x)*sin(eu_y)*cos(eu_z); sin(eu_x)*cos(eu_z)+cos(eu_x)*sin(eu_y)*sin(eu_z); cos(eu_x)*cos(eu_y)];
% R is 1x9

== matlab function controller_v10/Adaptive Controller/attitude and thrust controller/Thrust Controller ==
  data: r input; F output size=1; r_dot input; r_dotdot input; R input; Omega input; rd input; rd_d input; rd_dd input; rd_ddd input; rd_dddd input; int_e input; mdl parameter; alt_e output size=1; ctr parameter
function [F, alt_e] = fcn(r, r_dot, r_dotdot, R, Omega, rd,rd_d,rd_dd,rd_ddd,rd_dddd, int_e, mdl, ctr)
%#codegen

%% init
R11 = R(1);
R12 = R(2);
R13 = R(3);
R21 = R(4);
R22 = R(5);
R23 = R(6);
R31 = R(7);
R32 = R(8);
R33 = R(9);


F = rd_dd(3) - ctr.gain.al1*( r_dot(3)-rd_d(3) ) - ctr.gain.al0*( r(3)-rd(3) );
% F = 0 - ctr.gain.al1*( r_dot(3)) - ctr.gain.al0*( r(3)-ctr.setpoint.z );
F = mdl.g + F + ctr.gain.ali*int_e(4);
F = F/R33;
F = max(min(F, mdl.g+4), mdl.g-3.0); % during hovering.

alt_e = -( r(3)-rd(3) )/R33;
% alt_e = -( r(3)- ctr.setpoint.z )/R33;
end
